simulink model "sumOfVarSIM"  (R2021a)
settings: Solver=VariableStepAuto  StartTime=0.0  StopTime=100  RelTol=1e-3
values from neighbouring files (symbols this model uses):
  setMean_RN_1 = 0    [sumOfVar.m]
  setMean_RN_2 = 0    [sumOfVar.m]
  setSeed_RN_1 = 1234    [sumOfVar.m]
  setSeed_RN_2 = 4321    [sumOfVar.m]
  setVar_RN_1 = 100    [sumOfVar.m]
  setVar_RN_2 = 256    [sumOfVar.m]
settings Model: Creator=personF  LastModifiedBy=personF

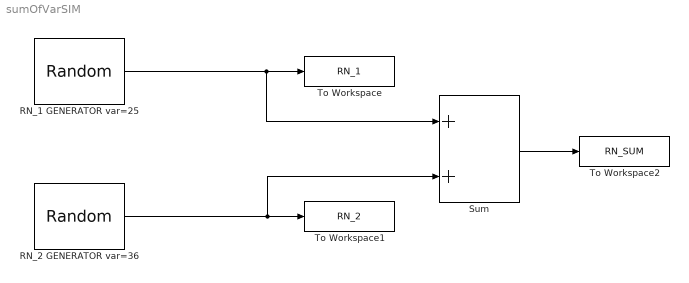
== system sumOfVarSIM ==
  RN_1 GENERATOR var=25 : RandomNumber  Mean=setMean_RN_1  Variance=setVar_RN_1  Seed=setSeed_RN_1  SampleTime=0.1
  RN_2 GENERATOR var=36 : RandomNumber  Mean=setMean_RN_2  Variance=setVar_RN_2  Seed=setSeed_RN_2  SampleTime=0.1
  Sum : Sum
  To Workspace : ToWorkspace  VariableName=RN_1  SampleTime=-1
  To Workspace1 : ToWorkspace  VariableName=RN_2  SampleTime=-1
  To Workspace2 : ToWorkspace  VariableName=RN_SUM  SampleTime=-1
  wires:
  RN_1 GENERATOR var=25/1 -> Sum/1, To Workspace/1
  RN_2 GENERATOR var=36/1 -> Sum/2, To Workspace1/1
  Sum/1 -> To Workspace2/1
